simulink library "dspmtrx2"  (Simulink 3.00)
libraries: dspmtrx2 x1
settings Model: Creator=szlotkin  LastModifiedBy=don

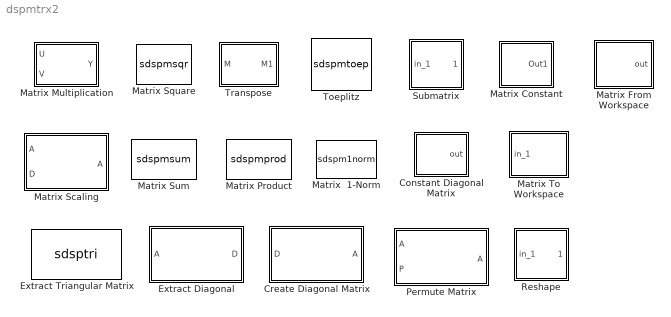
== system dspmtrx2 ==
  Constant Diagonal Matrix : Subsystem  mask(Constant Diagonal Matrix){n=3, q=1}
      mask prompts: n "Number of rows in matrix:"; q "Constant(s) along diagonal:"
      mask help:
      | Generate a full, diagonal matrix having elements specified by a vector
      | constant.  For a scalar constant, all diagonal elements will be identical.  To generate a diagonal scaling vector, use a constant block.
      mask init:
      | [a,x,y] = dspblkdiag(n,q);
      mask Help: web(dspbhelp);
      mask Display: plot(x,y)
  Create Diagonal Matrix : Subsystem  mask(Create Diagonal Matrix){}
      mask help: Convert a vector of diagonal elements to a full matrix.
      mask init:
      | ncols = -1;
      | mode = 1;
      | x = [.58 .87 .87 .58 .58 NaN 0.45 0.12 NaN 0.525 0.525 0.475 0.475 0.525 0.525 0.565 0.525 ];
      | y = [ 0.2 0.2 0.8 0.8 0.2 NaN 0.2 0.8 NaN 0.435 0.475 0.475 0.525 0.525 0.565 0.5 0.435 ];
      mask Help: web(dspbhelp);
      mask Display: plot(x,y)
  Extract Diagonal : Subsystem  mask(Extract Diagonal){ncols=-1}
      mask prompts: ncols "Number of columns in A (-1 for square):"
      mask help: Extract the main diagonal of a full matrix.
      mask init:
      | mode = 2;
      | x = [.58 .87 NaN 0.12 0.45 0.45 0.12 0.12 NaN 0.525 0.525 0.475 0.475 0.525 0.525 0.565 0.525 ];
      | y = [ 0.8 0.2 NaN 0.2 0.2 0.8 0.8 0.2 NaN 0.435 0.475 0.475 0.525 0.525 0.565 0.5 0.435 ];
      mask Help: web(dspbhelp);
      mask Display: plot(x,y)
  Extract Triangular Matrix : S-Function  FunctionName=sdsptri  Parameters=ncols,fcn  PortCounts=[]  SFunctionModules=''  mask(Extract Triangular Matrix){fcn=Upper, ncols=5}
      mask prompts: fcn "Extract:"; ncols "Number of columns in A:"
      mask help: Extract upper or lower triangular part of input matrix.
      mask init:
      | [s,x,y] = dspblktri(fcn);
      mask Help: web(dspbhelp);
      mask StyleString: popup(Upper|Lower),edit
      mask Display:
      | plot(x,y);
      | port_label('input',1,'A');
      | port_label('output',1,s);
  Matrix Constant : Subsystem  mask(Matrix Constant){M=rand(3,3)}
      mask prompts: M "Matrix:"
      mask help: Generate a constant matrix.
      mask init:
      | M2=M; s=size(M2);
      | if length(s)>2,
      |   s2=prod(s(2:end));
      |   M2=reshape(M2,s(1),s2);
      |   s=[s(1) s2];
      | end
      | s=sprintf('%dx%d',s(1),s(2));
      mask Help: web(dspbhelp);
      mask Display:
      | plot(0,0,100,100,
      | [20 10 10 20],[90 90 10 10],[84 96 96 84],[90 90 10 10]);
      | disp(s);
  Matrix From Workspace : Subsystem  mask(Matrix From Workspace){U=rand(3,3,5), Ts=1}
      mask prompts: U "3-D array (3rd dim spans time):"; Ts "Sample Time"
      mask help: Interpolate workspace array of time and matrix input values.
      mask init:
      | [M,N,P]=size(U);
      | dispstr=sprintf('%dx%dx%d',M,N,P);
      | s.time=[]; s.signals.values=reshape(U,M*N,P).';
      mask Help: web(dspbhelp);
      mask Display:
      | plot(0,0,100,100,
      | [20 10 10 20],[90 90 10 10],[84 96 96 84],[90 90 10 10]);
      | disp(dispstr);
  Matrix Multiplication : Subsystem  mask(Matrix Multiplication){Asize=[2 2], Bcols=2}
      mask prompts: Asize "Size of U, [rows cols]:"; Bcols "Number of columns in V:"
      mask help: Multiply two matrices.
      mask Help: web(dspbhelp);
      mask Display: disp(' U * V')
  Matrix Product : S-Function  FunctionName=sdspmprod  Parameters=Cols,Dim  PortCounts=[]  SFunctionModules=''  mask(Matrix Product){Dim=Columns, Cols=3}
      mask prompts: Dim "Multiply along:"; Cols "Number of columns in input:"
      mask help: Product of matrix elements along the row or column dimension.
      mask init:
      | if (Dim==1), str='Row\nProduct';
      | else str='Column\nProduct';
      | end
      mask Help: web(dspbhelp);
      mask StyleString: popup(Rows|Columns),edit
      mask Display: disp(str);
  Matrix Scaling : Subsystem  mask(Matrix Scaling){mode=Scale Rows (D*A), cols=1}
      mask prompts: cols "Number of columns in A:"
      mask help: Scale the columns or rows of a matrix A by the elements of a vector D. This is equivalent to multiplying a full matrix (A) by a diagonal (D), and vice-versa.
      mask init:
      | if mode==1, s='Scale\nRows'; else s='Scale\nColumns'; end
      mask Help: web(dspbhelp);
      mask StyleString: popup(Scale Rows (D*A)|Scale Columns (A*D)),edit
      mask Display: disp(s);
  Matrix Square : S-Function  FunctionName=sdspmsqr  Parameters=Acols  PortCounts=[]  SFunctionModules=''  mask(Matrix Square){Acols=3}
      mask prompts: Acols "Number of columns in input:"
      mask help: Compute the matrix square, U' * U. May be used with row and column input vectors to compute efficient outer and inner products. Hermitian transpose is performed for complex inputs.
      mask Help: web(dspbhelp);
      mask Display: disp('U'' * U')
  Matrix Sum : S-Function  FunctionName=sdspmsum  Parameters=Cols,Dim  PortCounts=[]  SFunctionModules=''  mask(Matrix Sum){Dim=Columns, Cols=3}
      mask prompts: Dim "Sum along:"; Cols "Number of columns in input:"
      mask help: Sum of matrix elements along the row or column dimension.
      mask init:
      | if (Dim==1), str='Row\nSum';
      | else str='Column\nSum';
      | end
      mask Help: web(dspbhelp);
      mask StyleString: popup(Rows|Columns),edit
      mask Display: disp(str);
  Matrix To Workspace : Subsystem  mask(Matrix To Workspace){matname=yout, maxrows=1000, deci=1, matsiz=[3 3]}
      mask prompts: matname "Array name:"; maxrows "Maximum number of matrices:"; deci "Decimation factor:"; matsiz "Matrix size:"
      mask help: Write a matrix signal into the workspace, storing the resulting time-sequence as a 3-D array with time running along the third dimension.
      mask Help: web(dspbhelp);
      mask Display: disp(matname)
  Matrix  1-Norm : S-Function  FunctionName=sdspm1norm  Parameters=Cols  PortCounts=[]  SFunctionModules=''  mask(Matrix 1-Norm){Cols=-1}
      mask prompts: Cols "Number of columns in input (-1 for square):"
      mask help: Compute the matrix 1-norm, which is the largest column sum of absolute values.
      mask Help: web(dspbhelp);
      mask Display: disp('Matrix\n1-Norm')
  Permute Matrix : Subsystem  mask(Permute Matrix){mode=Columns, errmode=Clip Index, cols=1}
      mask prompts: mode "Permute:"; errmode "Invalid Permutation Index:"; cols "Number of columns in A:"
      mask help: Permute the rows or columns of a matrix or vector A, based on a vector P of integer-valued permutation indices.
      mask Help: web(dspbhelp);
      mask StyleString: popup(Rows|Columns),popup(Clip Index|Clip and Warn|Generate Error),edit
      mask Display: disp(['Permute\n' &1])
  Reshape : Subsystem  mask(Reshape){Asiz=[2 2]}
      mask prompts: Asiz "New matrix size:"
      mask help: Reshape a vector or matrix to have size M-by-N. Output a new matrix whose elements are taken columnwise from the input. An error results if the input does not have M*N elements.
      mask init:
      | if ~exist('Asiz') | ~isequal(size(Asiz), [1 2]),
      |   s = '? ? ?';
      |   error('Matrix size must be a 2 element row vector');
      | else
      |   s=sprintf('%dx%d', Asiz);
      | end
      mask Help: web(dspbhelp);
      mask Display:
      | plot(0,0,100,100,
      | [20 10 10 20],[90 90 10 10],
      | [84 96 96 84],[90 90 10 10]);
      | disp(s);
  Submatrix : Subsystem  mask(Submatrix){siz=[3 3], expr={1:2, 2:3}}
      mask prompts: siz "Input matrix size, [rows cols]:"; expr "Index expression (cell-array):"
      mask help: Return a selected portion of a matrix signal. The submatrix is specified by a cell-array containing a comma-separated MATLAB indexing expression, expr, such that y=u(expr{:}). (The "end" keyword and lone colon operators are not supported.)
      mask init:
      | x1=[.2 .1 .1 .2 NaN .825 .925 .925 .825];
      | y1=[.9 .9 .1 .1 NaN .9 .9 .1 .1];
      | S=8; t=(0:S)'/S*2*pi; a=0.05;
      | x=a*cos(t);y=a*sin(t);
      | xc=x*ones(1,9) + ones(size(t))*[.3 .3 .3 .5 .5 .5 .7 .7 .7];
      | yc=y*ones(1,9) + ones(size(t))*[.25 .5 .75 .25 .5 .75 .25 .5 .75];
      | xi=[.4 .8 .8 .4 .4]; yi=[.375 .375 .875 .875 .375];
      | nele=prod(siz); idx=reshape(1:nele,siz);
      | idx=idx(expr{:}); idx=idx(:);
      mask Help: web(dspbhelp);
      mask Display: plot(x1,y1,xc,yc,xi,yi);
  Toeplitz : S-Function  FunctionName=sdspmtoep  Parameters=Symmetric  PortCounts=[]  SFunctionModules=''  mask(Toeplitz){Symmetric=on}
      mask help: Generate a Toeplitz matrix having input Col as its first column and Row as its first row. If Symmetric is checked, a symmetric (or Hermitian) Toeplitz matrix is generated with Row as its first row.
      mask init:
      | if (Symmetric==1)
      |   p1 = 1; L1 = 'Row';
      |   p2 = 1;  L2 = 'Row';
      | else
      |   p1 = 1;  L1 = 'Col';
      |   p2 = 2;  L2 = 'Row';
      | end
      | 
      | xm=.25 +.8*[0.25 0.1625 0.1625 0.25 NaN 0.7875 0.8875 0.8875 0.7875 NaN 0.25 0.75 NaN 0.4125 0.75 NaN 0.5875 0.75 NaN 0.25 0.5875 NaN 0.25 0.4125];
      | ym=[.9 .9 .1 .1 NaN .9 .9 .1 .1 NaN .8 .2 NaN .8 .4 NaN .8 .6 NaN .6 .2 NaN .4 .2];
      mask Help: web(dspbhelp);
      mask Display:
      | plot(xm,ym);
      | port_label('input', p1, L1);
      | port_label('input', p2, L2);
  Transpose : Subsystem  mask(Transpose){Asize=3, Hermitian=off}
      mask prompts: Asize "Number of columns in input:"
      mask help: Compute the matrix transpose.
      mask init:
      | if(Hermitian==1),  str = ' U ''';
      | else,                    str = ' U.''';
      | end
      mask Help: web(dspbhelp);
      mask Display: disp(str)

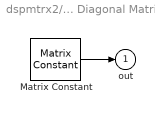
== system dspmtrx2/Constant Diagonal Matrix ==
  Matrix Constant : dspmtrx2/Matrix Constant  M=a
  out : Outport  Port=1  InitialOutput=0
  wires:
  Matrix Constant/1 -> out/1

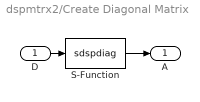
== system dspmtrx2/Create Diagonal Matrix ==
  D : Inport  Port=1  PortWidth=-1  SampleTime=-1  DataType=auto
      settings: SignalType=auto
  S-Function : S-Function  FunctionName=sdspdiag  Parameters=ncols,mode  PortCounts=[]  SFunctionModules=''
  A : Outport  Port=1
  wires:
  D/1 -> S-Function/1
  S-Function/1 -> A/1

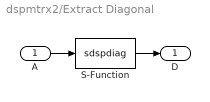
== system dspmtrx2/Extract Diagonal ==
  A : Inport  Port=1  PortWidth=-1  SampleTime=-1  DataType=auto
      settings: SignalType=auto
  S-Function : S-Function  FunctionName=sdspdiag  Parameters=ncols,mode  PortCounts=[]  SFunctionModules=''
  D : Outport  Port=1
  wires:
  A/1 -> S-Function/1
  S-Function/1 -> D/1

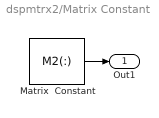
== system dspmtrx2/Matrix Constant ==
  Matrix  Constant : Constant  Value=M2(:)
  Out1 : Outport  Port=1  InitialOutput=0
  wires:
  Matrix  Constant/1 -> Out1/1

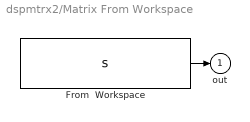
== system dspmtrx2/Matrix From Workspace ==
  From  Workspace : FromWorkspace  VariableName=s  SampleTime=Ts  Interpolate=off  HoldFinalValue=off
  out : Outport  Port=1  InitialOutput=0
  wires:
  From  Workspace/1 -> out/1

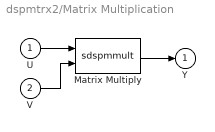
== system dspmtrx2/Matrix Multiplication ==
  U : Inport  Port=1  PortWidth=-1  SampleTime=-1  DataType=auto
      settings: SignalType=auto
  V : Inport  Port=2  PortWidth=-1  SampleTime=-1  DataType=auto
      settings: SignalType=auto
  Matrix Multiply : S-Function  FunctionName=sdspmmult  Parameters=Asize,Bcols  PortCounts=[]  SFunctionModules=''
  Y : Outport  Port=1  InitialOutput=0
  wires:
  U/1 -> Matrix Multiply/1
  V/1 -> Matrix Multiply/2
  Matrix Multiply/1 -> Y/1

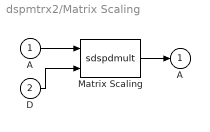
== system dspmtrx2/Matrix Scaling ==
  A : Inport  Port=1  PortWidth=-1  SampleTime=-1  DataType=auto
      settings: SignalType=auto
  D : Inport  Port=2  PortWidth=-1  SampleTime=-1  DataType=auto
      settings: SignalType=auto
  Matrix Scaling : S-Function  FunctionName=sdspdmult  Parameters=mode,cols  PortCounts=[]  SFunctionModules=''
  " A" : Outport  Port=1  InitialOutput=0
  wires:
  D/1 -> Matrix Scaling/2
  A/1 -> Matrix Scaling/1
  Matrix Scaling/1 -> " A"/1

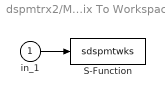
== system dspmtrx2/Matrix To Workspace ==
  in_1 : Inport  Port=1  PortWidth=-1  SampleTime=-1  DataType=auto
      settings: SignalType=auto
  S-Function : S-Function  FunctionName=sdspmtwks  Parameters=matname,maxrows,deci,matsiz  PortCounts=[]  SFunctionModules=''
  wires:
  in_1/1 -> S-Function/1

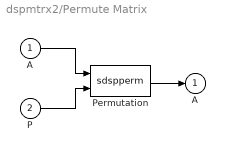
== system dspmtrx2/Permute Matrix ==
  A : Inport  Port=1  PortWidth=-1  SampleTime=-1  DataType=auto
      settings: SignalType=auto
  P : Inport  Port=2  PortWidth=-1  SampleTime=-1  DataType=auto
      settings: SignalType=auto
  Permutation : S-Function  FunctionName=sdspperm  Parameters=mode,errmode,cols  PortCounts=[]  SFunctionModules=''
  " A" : Outport  Port=1  InitialOutput=0
  wires:
  Permutation/1 -> " A"/1
  P/1 -> Permutation/2
  A/1 -> Permutation/1

== system dspmtrx2/Reshape ==
  in_1 : Inport  Port=1  PortWidth=-1  SampleTime=-1  DataType=auto
      settings: SignalType=auto
  out_1 : Outport  Port=1  InitialOutput=0
  wires:
  in_1/1 -> out_1/1

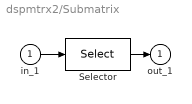
== system dspmtrx2/Submatrix ==
  in_1 : Inport  Port=1  PortWidth=-1  SampleTime=-1  DataType=auto
      settings: SignalType=auto
  Selector : Selector  Elements=idx  InputPortWidth=nele
  out_1 : Outport  Port=1  InitialOutput=0
  wires:
  in_1/1 -> Selector/1
  Selector/1 -> out_1/1

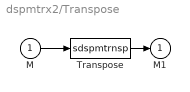
== system dspmtrx2/Transpose ==
  M : Inport  Port=1  PortWidth=-1  SampleTime=-1  DataType=auto
      settings: SignalType=auto
  Transpose : S-Function  FunctionName=sdspmtrnsp  Parameters=Asize, Hermitian  PortCounts=[]  SFunctionModules=''
  M1 : Outport  Port=1  InitialOutput=0
  wires:
  M/1 -> Transpose/1
  Transpose/1 -> M1/1
